simulink model "FOC_sensored"  (R2026a)
settings: Solver=VariableStepAuto  StopTime=3  MaxStep=1e-4  RelTol=1e-4
undefined symbols (not defined in the file): Encoder_resolution, G_filt_back_den_current, G_filt_back_num_current, G_filt_cont_den_current, G_filt_cont_num_current, G_filt_disc_emu_back_den_current, G_filt_disc_emu_back_num_current, G_filt_disc_emu_forw_den_current, G_filt_disc_emu_forw_num_current, G_filt_forw_den_current, G_filt_forw_num_current, In, J, Kr_cont_current, Kr_cont_speed, Kr_direct_back_current, Kr_direct_forw_current, Ld, Lq, Ls, Mn, nn, pp, Psir, T_speed_feedback, Ti_cont_current, Ti_cont_speed, Ti_direct_back_current, Ti_direct_forw_current, Ts_current, Udc
libraries: fl_lib x43, nesl_utility x37, ee_lib x18, eeTransforms x12, slpidlib x5
(part 1 of 2)
settings Model: Creator=LukaPravica  LastModifiedBy=Rio
settings SimscapeCC: ExplicitSolverDiagnosticOptions=none  SimscapeNominalValues="[{\"value\":\"1\",\"unit\":\"A\"},{\"value\":\"1\",\"unit\":\"bar\"},{\"value\":\"1\",\"unit\":\"cm^2\"},{\"value\":\"1\",\"unit\":\"cm^3/s\"},{\"value\":\"1\",\"unit\":\"kJ/kg\"},{\"value\":\"1\",\"unit\":\"kW\"},{\"value\":\"1\",\"unit\":\"l\"},{\"value\":\"1\",\"unit\":\"N\"},{\"value\":\"1\",\"unit\":\"N*m\"},{\"value\":\"1\",\"unit\":\"V\"}]"  SimscapeLogType=none  SimscapeLogDataHistory=5000.0

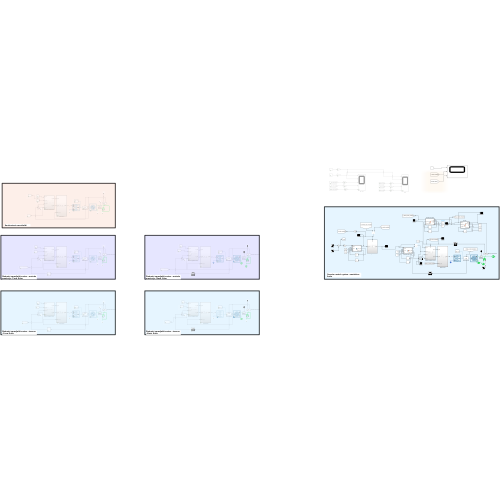
[thumbnail: Simulink's stored preview of the top-level diagram]
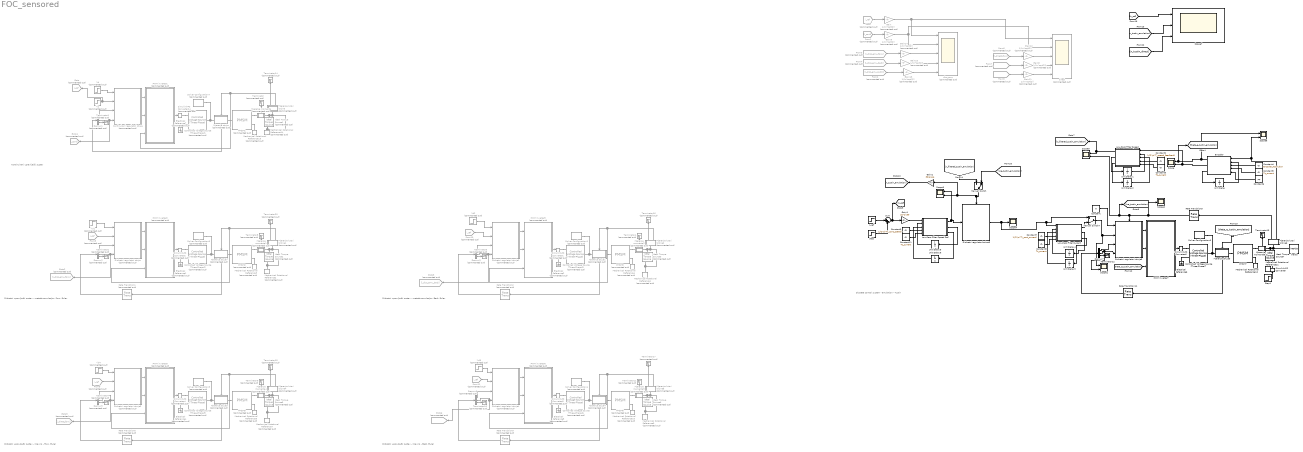
== system FOC_sensored ==
  note: Diskretni upravljački sustav - metoda emulacije - Forw. Euler
  note: Kontinuirani upravljački sustav
  note: Diskretni upravljački sustav - metoda emulacije - Back. Euler
  note: Diskretni upravljački sustav - izravno - Forw. Euler
  note: Diskretni upravljački sustav - izravno - Back. Euler
  note: Discrete control system - emulation - Tustin
  *id{,1..2,4..5} (5 alike) : Step  Commented=on  FinalValue=0  SampleTime=0
  *iq : Step  Commented=on  Time=0.001  FinalValue=In*sqrt(2)  SampleTime=0
  Constant : Constant  Value=0  SampleTime=Ts_current
  Constant{3,5,8,11} (4 alike) : Constant  Value=Ts_current  SampleTime=Ts_current
  Constant2 : Constant  Value=1/(2*pi*T_speed_feedback)  SampleTime=Ts_current
  Constant4 : Constant  Value=Encoder_resolution  SampleTime=Ts_current
  Constant6 : Constant  Value=pp  SampleTime=Ts_current
  Constant7 : Constant  Value=1/(2*pi*Ti_cont_current)  SampleTime=Ts_current
  Constant9 : Constant  Value=1/(2*pi*Ti_cont_speed)  SampleTime=Ts_current
  Controlled Voltage Source (Three-Phase){1..3,5..6} (5 alike) : ee_lib/Sources/Controlled Voltage Source (Three-Phase)  Commented=on  input_option=ee.enum.inputType.instantaneous  FRated=60 Hz
  Controlled Voltage Source (Three-Phase)7 : ee_lib/Sources/Controlled Voltage Source (Three-Phase)  input_option=ee.enum.inputType.instantaneous  FRated=60 Hz
  Demux{1..3,5..6} (5 alike) : Demux  Commented=on  Outputs=3
  Demux7 : Demux  Outputs=3
  Diskretni regulator brzine5 : Subsystem
      settings: PortSchema="{\"entries\":[{\"content\":{\"sides\":[{\"content\":{\"connectorIds\":[\"In1\"]},\"type\":\"ConnectorPlacement.EquallySpacedRectSide\",\"uuid\":\"a9765fbc-5a4d-474e-be8d-5c320c5f07ca\"},{\"content\":{\"connectorIds\":[\"Out1\"],\"side\":\"RIGHT\"},\"type\":\"ConnectorPlacement.EquallySpacedRectSide\",\"uuid\":\"d113e0d0-4772-4877-8676-69342ee8f64f\"},{\"content\":{\"connectorIds\":[\"In2\"],\"side\":\"TOP\"},\"type\":\"ConnectorPlacement.EquallySpacedRectSide\",\"uuid\":\"4ca0dc59-fd41-4846-82a7-6904cf53659d\"}]},\"type\":\"ConnectorPlacement.EquallySpacedConnector\",\"uuid\":\"7fdfac1a-ebdc-43ed-9adb-be729266989d\"}],\"packageUris\":[\"http://schema.mathworks.com/mf0/Connector/R2020b\"],\"version\":\"1.0\"}"
  Diskretni regulatori struje : Subsystem  Commented=on
  Diskretni regulatori struje1 : Subsystem  Commented=on
  Diskretni regulatori struje3 : Subsystem  Commented=on
  Diskretni regulatori struje4 : Subsystem  Commented=on
  Diskretni regulatori struje5 : Subsystem
      settings: PortSchema="{\"entries\":[{\"content\":{\"sides\":[{\"content\":{\"connectorIds\":[\"In1\",\"In2\",\"In3\",\"In4\"]},\"type\":\"ConnectorPlacement.EquallySpacedRectSide\",\"uuid\":\"d3a62493-f7c6-444f-9476-25937989f6ea\"},{\"content\":{\"connectorIds\":[\"Out1\",\"Out2\"],\"side\":\"RIGHT\"},\"type\":\"ConnectorPlacement.EquallySpacedRectSide\",\"uuid\":\"ca5c9823-b9be-4b72-ab87-a2cad855a0f6\"},{\"content\":{\"connectorIds\":[\"In5\"],\"side\":\"TOP\"},\"type\":\"ConnectorPlacement.EquallySpacedRectSide\",\"uuid\":\"496b345e-fed9-4adb-95d9-010d07f11d94\"}]},\"type\":\"ConnectorPlacement.EquallySpacedConnector\",\"uuid\":\"9eb14200-6fae-48ad-9447-ab4bb77ea536\"}],\"packageUris\":[\"http://schema.mathworks.com/mf0/Connector/R2020b\"],\"version\":\"1.0\"}"
  Electrical Reference{1..2,4..5,7} (5 alike) : fl_lib/Electrical/Electrical Elements/Electrical Reference  Commented=on
  Electrical Reference6 : fl_lib/Electrical/Electrical Elements/Electrical Reference
  Encoder : MATLAB Function  TreatAsAtomicUnit=on
  From{,8..11} (5 alike) : From  Commented=on  GotoTag=i_ref  TagVisibility=global
  From1 : From  Commented=on  GotoTag=i_cont
  From2 : From  Commented=on  GotoTag=i_disc_emu_tustin
  From3 : From  Commented=on  GotoTag=i_disc_emu_forw
  From4 : From  Commented=on  GotoTag=i_disc_emu_back
  From5 : From  Commented=on  GotoTag=i_direct_tustin
  From6 : From  Commented=on  GotoTag=i_direct_forw
  From7 : From  Commented=on  GotoTag=i_direct_back
  Gain{,8..14} (8 alike) : Gain  Commented=on  Gain=1/(In*sqrt(2))
  Gain1 : Gain  Gain=pp*pi/30
  Gain2 : Gain  Gain=30/pi/pp
  Goto : Goto  Commented=on  GotoTag=i_ref  TagVisibility=global
  Goto1 : Goto  Commented=on  GotoTag=i_cont
  Goto2 : Goto  Commented=on  GotoTag=i_disc_emu_forw
  Goto3 : Goto  Commented=on  GotoTag=i_disc_emu_back
  Goto5 : Goto  Commented=on  GotoTag=i_direct_forw
  Goto6 : Goto  Commented=on  GotoTag=i_direct_back
  Ideal Torque Source{1..3,5..6} (5 alike) : fl_lib/Mechanical/Mechanical Sources/Ideal Torque Source  Commented=on
  Ideal Torque Source7 : fl_lib/Mechanical/Mechanical Sources/Ideal Torque Source
  Inertia : fl_lib/Mechanical/Rotational Elements/Inertia  inertia=J kg*m^2  num_ports=foundation.enum.numPorts2.one  w_specify=off  w_priority=High  w=0 rad/s  w_nominal_specify=off  w_nominal_value=1  w_nominal_unit=rad/s  t_specify=off  t_priority=None  t=0 N*m  t_nominal_specify=off  t_nominal_value=1  t_nominal_unit=N*m
  Kontinuirani regulatori struje : Subsystem  Commented=on
  Low-Pass Filter Current : MATLAB Function  TreatAsAtomicUnit=on
  Low-Pass Filter Speed : MATLAB Function  TreatAsAtomicUnit=on
  Low-Pass Filter Speed Ref : MATLAB Function  TreatAsAtomicUnit=on
  Manual Switch : ManualSwitch  CurrentSetting=0
  Manual Switch7 : ManualSwitch  CurrentSetting=0
  Mechanical Rotational Reference{1..4,7..10,14..15} (10 alike) : fl_lib/Mechanical/Rotational Elements/Mechanical Rotational Reference  Commented=on
  Mechanical Rotational Reference11 : fl_lib/Mechanical/Rotational Elements/Mechanical Rotational Reference
  Mechanical Rotational Reference12 : fl_lib/Mechanical/Rotational Elements/Mechanical Rotational Reference
  Mjerenje momenta : Subsystem  Commented=on
      settings: PortSchema="{\"entries\":[{\"content\":{\"sides\":[{\"content\":{\"connectorIds\":[\"LConn1\"]},\"type\":\"ConnectorPlacement.EquallySpacedRectSide\",\"uuid\":\"6fa7c16c-6de5-49c8-bc22-739ef8014510\"},{\"content\":{\"connectorIds\":[\"RConn1\"],\"side\":\"RIGHT\"},\"type\":\"ConnectorPlacement.EquallySpacedRectSide\",\"uuid\":\"6cbb3fe1-95dc-4f03-932b-ab8cb637a208\"},{\"content\":{\"connectorIds\":[\"Out1\"],\"side\":\"TOP\"},\"type\":\"ConnectorPlacement.EquallySpacedRectSide\",\"uuid\":\"35a7ae71-901f-47d3-ac0b-d21c2464290d\"}]},\"type\":\"ConnectorPlacement.EquallySpacedConnector\",\"uuid\":\"03aa7740-1fdb-47bb-9a21-844669f6bcda\"}],\"packageUris\":[\"http://schema.mathworks.com/mf0/Connector/R2020b\"],\"version\":\"1.0\"}"
      mask Display: disp('trq')
  Mjerenje momenta1 : Subsystem  Commented=on
      settings: PortSchema="{\"entries\":[{\"content\":{\"sides\":[{\"content\":{\"connectorIds\":[\"LConn1\"]},\"type\":\"ConnectorPlacement.EquallySpacedRectSide\",\"uuid\":\"6fa7c16c-6de5-49c8-bc22-739ef8014510\"},{\"content\":{\"connectorIds\":[\"RConn1\"],\"side\":\"RIGHT\"},\"type\":\"ConnectorPlacement.EquallySpacedRectSide\",\"uuid\":\"6cbb3fe1-95dc-4f03-932b-ab8cb637a208\"},{\"content\":{\"connectorIds\":[\"Out1\"],\"side\":\"TOP\"},\"type\":\"ConnectorPlacement.EquallySpacedRectSide\",\"uuid\":\"35a7ae71-901f-47d3-ac0b-d21c2464290d\"}]},\"type\":\"ConnectorPlacement.EquallySpacedConnector\",\"uuid\":\"03aa7740-1fdb-47bb-9a21-844669f6bcda\"}],\"packageUris\":[\"http://schema.mathworks.com/mf0/Connector/R2020b\"],\"version\":\"1.0\"}"
      mask Display: disp('trq')
  Mjerenje momenta2 : Subsystem  Commented=on
      settings: PortSchema="{\"entries\":[{\"content\":{\"sides\":[{\"content\":{\"connectorIds\":[\"LConn1\"]},\"type\":\"ConnectorPlacement.EquallySpacedRectSide\",\"uuid\":\"6fa7c16c-6de5-49c8-bc22-739ef8014510\"},{\"content\":{\"connectorIds\":[\"RConn1\"],\"side\":\"RIGHT\"},\"type\":\"ConnectorPlacement.EquallySpacedRectSide\",\"uuid\":\"6cbb3fe1-95dc-4f03-932b-ab8cb637a208\"},{\"content\":{\"connectorIds\":[\"Out1\"],\"side\":\"TOP\"},\"type\":\"ConnectorPlacement.EquallySpacedRectSide\",\"uuid\":\"35a7ae71-901f-47d3-ac0b-d21c2464290d\"}]},\"type\":\"ConnectorPlacement.EquallySpacedConnector\",\"uuid\":\"03aa7740-1fdb-47bb-9a21-844669f6bcda\"}],\"packageUris\":[\"http://schema.mathworks.com/mf0/Connector/R2020b\"],\"version\":\"1.0\"}"
      mask Display: disp('trq')
  Mjerenje momenta4 : Subsystem  Commented=on
      settings: PortSchema="{\"entries\":[{\"content\":{\"sides\":[{\"content\":{\"connectorIds\":[\"LConn1\"]},\"type\":\"ConnectorPlacement.EquallySpacedRectSide\",\"uuid\":\"6fa7c16c-6de5-49c8-bc22-739ef8014510\"},{\"content\":{\"connectorIds\":[\"RConn1\"],\"side\":\"RIGHT\"},\"type\":\"ConnectorPlacement.EquallySpacedRectSide\",\"uuid\":\"6cbb3fe1-95dc-4f03-932b-ab8cb637a208\"},{\"content\":{\"connectorIds\":[\"Out1\"],\"side\":\"TOP\"},\"type\":\"ConnectorPlacement.EquallySpacedRectSide\",\"uuid\":\"35a7ae71-901f-47d3-ac0b-d21c2464290d\"}]},\"type\":\"ConnectorPlacement.EquallySpacedConnector\",\"uuid\":\"03aa7740-1fdb-47bb-9a21-844669f6bcda\"}],\"packageUris\":[\"http://schema.mathworks.com/mf0/Connector/R2020b\"],\"version\":\"1.0\"}"
      mask Display: disp('trq')
  Mjerenje momenta5 : Subsystem  Commented=on
      settings: PortSchema="{\"entries\":[{\"content\":{\"sides\":[{\"content\":{\"connectorIds\":[\"LConn1\"]},\"type\":\"ConnectorPlacement.EquallySpacedRectSide\",\"uuid\":\"6fa7c16c-6de5-49c8-bc22-739ef8014510\"},{\"content\":{\"connectorIds\":[\"RConn1\"],\"side\":\"RIGHT\"},\"type\":\"ConnectorPlacement.EquallySpacedRectSide\",\"uuid\":\"6cbb3fe1-95dc-4f03-932b-ab8cb637a208\"},{\"content\":{\"connectorIds\":[\"Out1\"],\"side\":\"TOP\"},\"type\":\"ConnectorPlacement.EquallySpacedRectSide\",\"uuid\":\"35a7ae71-901f-47d3-ac0b-d21c2464290d\"}]},\"type\":\"ConnectorPlacement.EquallySpacedConnector\",\"uuid\":\"03aa7740-1fdb-47bb-9a21-844669f6bcda\"}],\"packageUris\":[\"http://schema.mathworks.com/mf0/Connector/R2020b\"],\"version\":\"1.0\"}"
      mask Display: disp('trq')
  Mjerenje momenta6 : Subsystem
      settings: PortSchema="{\"entries\":[{\"content\":{\"sides\":[{\"content\":{\"connectorIds\":[\"LConn1\"]},\"type\":\"ConnectorPlacement.EquallySpacedRectSide\",\"uuid\":\"6fa7c16c-6de5-49c8-bc22-739ef8014510\"},{\"content\":{\"connectorIds\":[\"RConn1\"],\"side\":\"RIGHT\"},\"type\":\"ConnectorPlacement.EquallySpacedRectSide\",\"uuid\":\"6cbb3fe1-95dc-4f03-932b-ab8cb637a208\"},{\"content\":{\"connectorIds\":[\"Out1\"],\"side\":\"TOP\"},\"type\":\"ConnectorPlacement.EquallySpacedRectSide\",\"uuid\":\"35a7ae71-901f-47d3-ac0b-d21c2464290d\"}]},\"type\":\"ConnectorPlacement.EquallySpacedConnector\",\"uuid\":\"03aa7740-1fdb-47bb-9a21-844669f6bcda\"}],\"packageUris\":[\"http://schema.mathworks.com/mf0/Connector/R2020b\"],\"version\":\"1.0\"}"
      mask Display: disp('trq')
  Mjerenje kuta i brzine : Subsystem  Commented=on
      mask Display: disp('w,a')
  Mjerenje kuta i brzine1 : Subsystem  Commented=on
      mask Display: disp('w,a')
  Mjerenje kuta i brzine2 : Subsystem  Commented=on
      mask Display: disp('w,a')
  Mjerenje kuta i brzine4 : Subsystem  Commented=on
      mask Display: disp('w,a')
  Mjerenje kuta i brzine5 : Subsystem  Commented=on
      mask Display: disp('w,a')
  Mjerenje kuta i brzine6 : Subsystem
      mask Display: disp('w,a')
  Mjerenje struje : Subsystem  Commented=on
      settings: PortSchema="{\"entries\":[{\"content\":{\"sides\":[{\"content\":{\"connectorIds\":[\"LConn1\"]},\"type\":\"ConnectorPlacement.EquallySpacedRectSide\",\"uuid\":\"6fa7c16c-6de5-49c8-bc22-739ef8014510\"},{\"content\":{\"connectorIds\":[\"RConn1\"],\"side\":\"RIGHT\"},\"type\":\"ConnectorPlacement.EquallySpacedRectSide\",\"uuid\":\"6cbb3fe1-95dc-4f03-932b-ab8cb637a208\"},{\"content\":{\"connectorIds\":[\"In1\"],\"side\":\"TOP\"},\"type\":\"ConnectorPlacement.EquallySpacedRectSide\",\"uuid\":\"35a7ae71-901f-47d3-ac0b-d21c2464290d\"},{\"content\":{\"connectorIds\":[\"Out1\"],\"side\":\"BOTTOM\"},\"type\":\"ConnectorPlacement.EquallySpacedRectSide\",\"uuid\":\"976aabfd-697c-47ce-8be7-acff7370fc8c\"}]},\"type\":\"ConnectorPlacement.EquallySpacedConnector\",\"uuid\":\"03aa7740-1fdb-47bb-9a21-844669f6bcda\"}],\"packageUris\":[\"http://schema.mathworks.com/mf0/Connector/R2020b\"],\"version\":\"1.0\"}"
      mask Display: disp('vi abc')
  Mjerenje struje1 : Subsystem  Commented=on
      settings: PortSchema="{\"entries\":[{\"content\":{\"sides\":[{\"content\":{\"connectorIds\":[\"LConn1\"]},\"type\":\"ConnectorPlacement.EquallySpacedRectSide\",\"uuid\":\"6fa7c16c-6de5-49c8-bc22-739ef8014510\"},{\"content\":{\"connectorIds\":[\"RConn1\"],\"side\":\"RIGHT\"},\"type\":\"ConnectorPlacement.EquallySpacedRectSide\",\"uuid\":\"6cbb3fe1-95dc-4f03-932b-ab8cb637a208\"},{\"content\":{\"connectorIds\":[\"In1\"],\"side\":\"TOP\"},\"type\":\"ConnectorPlacement.EquallySpacedRectSide\",\"uuid\":\"35a7ae71-901f-47d3-ac0b-d21c2464290d\"},{\"content\":{\"connectorIds\":[\"Out1\"],\"side\":\"BOTTOM\"},\"type\":\"ConnectorPlacement.EquallySpacedRectSide\",\"uuid\":\"976aabfd-697c-47ce-8be7-acff7370fc8c\"}]},\"type\":\"ConnectorPlacement.EquallySpacedConnector\",\"uuid\":\"03aa7740-1fdb-47bb-9a21-844669f6bcda\"}],\"packageUris\":[\"http://schema.mathworks.com/mf0/Connector/R2020b\"],\"version\":\"1.0\"}"
      mask Display: disp('vi abc')
  Mjerenje struje3 : Subsystem  Commented=on
      settings: PortSchema="{\"entries\":[{\"content\":{\"sides\":[{\"content\":{\"connectorIds\":[\"LConn1\"]},\"type\":\"ConnectorPlacement.EquallySpacedRectSide\",\"uuid\":\"6fa7c16c-6de5-49c8-bc22-739ef8014510\"},{\"content\":{\"connectorIds\":[\"RConn1\"],\"side\":\"RIGHT\"},\"type\":\"ConnectorPlacement.EquallySpacedRectSide\",\"uuid\":\"6cbb3fe1-95dc-4f03-932b-ab8cb637a208\"},{\"content\":{\"connectorIds\":[\"In1\"],\"side\":\"TOP\"},\"type\":\"ConnectorPlacement.EquallySpacedRectSide\",\"uuid\":\"35a7ae71-901f-47d3-ac0b-d21c2464290d\"},{\"content\":{\"connectorIds\":[\"Out1\"],\"side\":\"BOTTOM\"},\"type\":\"ConnectorPlacement.EquallySpacedRectSide\",\"uuid\":\"976aabfd-697c-47ce-8be7-acff7370fc8c\"}]},\"type\":\"ConnectorPlacement.EquallySpacedConnector\",\"uuid\":\"03aa7740-1fdb-47bb-9a21-844669f6bcda\"}],\"packageUris\":[\"http://schema.mathworks.com/mf0/Connector/R2020b\"],\"version\":\"1.0\"}"
      mask Display: disp('vi abc')
  Mjerenje struje4 : Subsystem  Commented=on
      settings: PortSchema="{\"entries\":[{\"content\":{\"sides\":[{\"content\":{\"connectorIds\":[\"LConn1\"]},\"type\":\"ConnectorPlacement.EquallySpacedRectSide\",\"uuid\":\"6fa7c16c-6de5-49c8-bc22-739ef8014510\"},{\"content\":{\"connectorIds\":[\"RConn1\"],\"side\":\"RIGHT\"},\"type\":\"ConnectorPlacement.EquallySpacedRectSide\",\"uuid\":\"6cbb3fe1-95dc-4f03-932b-ab8cb637a208\"},{\"content\":{\"connectorIds\":[\"In1\"],\"side\":\"TOP\"},\"type\":\"ConnectorPlacement.EquallySpacedRectSide\",\"uuid\":\"35a7ae71-901f-47d3-ac0b-d21c2464290d\"},{\"content\":{\"connectorIds\":[\"Out1\"],\"side\":\"BOTTOM\"},\"type\":\"ConnectorPlacement.EquallySpacedRectSide\",\"uuid\":\"976aabfd-697c-47ce-8be7-acff7370fc8c\"}]},\"type\":\"ConnectorPlacement.EquallySpacedConnector\",\"uuid\":\"03aa7740-1fdb-47bb-9a21-844669f6bcda\"}],\"packageUris\":[\"http://schema.mathworks.com/mf0/Connector/R2020b\"],\"version\":\"1.0\"}"
      mask Display: disp('vi abc')
  Mjerenje struje5 : Subsystem
      settings: PortSchema="{\"entries\":[{\"content\":{\"sides\":[{\"content\":{\"connectorIds\":[\"LConn1\"]},\"type\":\"ConnectorPlacement.EquallySpacedRectSide\",\"uuid\":\"6fa7c16c-6de5-49c8-bc22-739ef8014510\"},{\"content\":{\"connectorIds\":[\"RConn1\"],\"side\":\"RIGHT\"},\"type\":\"ConnectorPlacement.EquallySpacedRectSide\",\"uuid\":\"6cbb3fe1-95dc-4f03-932b-ab8cb637a208\"},{\"content\":{\"connectorIds\":[\"In1\"],\"side\":\"TOP\"},\"type\":\"ConnectorPlacement.EquallySpacedRectSide\",\"uuid\":\"35a7ae71-901f-47d3-ac0b-d21c2464290d\"},{\"content\":{\"connectorIds\":[\"Out1\"],\"side\":\"BOTTOM\"},\"type\":\"ConnectorPlacement.EquallySpacedRectSide\",\"uuid\":\"976aabfd-697c-47ce-8be7-acff7370fc8c\"}]},\"type\":\"ConnectorPlacement.EquallySpacedConnector\",\"uuid\":\"03aa7740-1fdb-47bb-9a21-844669f6bcda\"}],\"packageUris\":[\"http://schema.mathworks.com/mf0/Connector/R2020b\"],\"version\":\"1.0\"}"
      mask Display: disp('vi abc')
  Mjerenje struje7 : Subsystem  Commented=on
      settings: PortSchema="{\"entries\":[{\"content\":{\"sides\":[{\"content\":{\"connectorIds\":[\"LConn1\"]},\"type\":\"ConnectorPlacement.EquallySpacedRectSide\",\"uuid\":\"6fa7c16c-6de5-49c8-bc22-739ef8014510\"},{\"content\":{\"connectorIds\":[\"RConn1\"],\"side\":\"RIGHT\"},\"type\":\"ConnectorPlacement.EquallySpacedRectSide\",\"uuid\":\"6cbb3fe1-95dc-4f03-932b-ab8cb637a208\"},{\"content\":{\"connectorIds\":[\"In1\"],\"side\":\"TOP\"},\"type\":\"ConnectorPlacement.EquallySpacedRectSide\",\"uuid\":\"35a7ae71-901f-47d3-ac0b-d21c2464290d\"},{\"content\":{\"connectorIds\":[\"Out1\"],\"side\":\"BOTTOM\"},\"type\":\"ConnectorPlacement.EquallySpacedRectSide\",\"uuid\":\"976aabfd-697c-47ce-8be7-acff7370fc8c\"}]},\"type\":\"ConnectorPlacement.EquallySpacedConnector\",\"uuid\":\"03aa7740-1fdb-47bb-9a21-844669f6bcda\"}],\"packageUris\":[\"http://schema.mathworks.com/mf0/Connector/R2020b\"],\"version\":\"1.0\"}"
      mask Display: disp('vi abc')
  PMSM1 : ee_lib/Electromechanical/Permanent Magnet/PMSM  Commented=on  port_option=ee.enum.threePhasePort.composite  winding_type=ee.enum.statorconnection.wye  machine_param=ee.enum.pmsm.parameterization.constant  nPolePairs=pp  pmflux_param=ee.enum.pmflux.fluxlinkage  pm_flux_linkage=Psir Wb  torque_constant=0.18 N*m/A  back_emf_constant=0.18 V/rpm  stator_param=ee.enum.statorparam.LdLqL0  Ld=Ls H  Lq=Ls H  idVec=[-200, 0, 200] A  iqVec=[-200, 0, 200] A  LdMatrix=0.0002 * ones(3, 3) H  LqMatrix=0.0002 * ones(3, 3) H  PmMatrix=0.1 * ones(3, 3) Wb  ktMatrix=0.18 * ones(3, 3) N*m/A  keMatrix=0.18 * ones(3, 3) V*s/rad  L0=(Ld+Lq)/2 H  Ls=0.0002 H  Lm=-0.00002 H  Ms=0.00002 H  Rs=Rs Ohm  zero_sequence=ee.enum.park.zerosequence.exclude  axes_param=ee.enum.rotorangle.daxis  loss_param=ee.enum.ironloss.none  losses_oc=[0, 0, 0] W  losses_sc=[0, 0, 0] W  f_losses=60 Hz  Isc_losses=95 A  J=J kg*m^2  lam=D N*m*s/rad  i_d_specify=off  i_d_priority=None  i_d=0 A  i_d_nominal_specify=off  i_d_nominal_value=1  i_d_nominal_unit=A  i_q_specify=off  i_q_priority=None  i_q=0 A  i_q_nominal_specify=off  i_q_nominal_value=1  i_q_nominal_unit=A  torque_specify=off  torque_priority=None  torque=0 N*m  torque_nominal_specify=off  torque_nominal_value=1  torque_nominal_unit=N*m  angular_velocity_specify=off  angular_velocity_priority=High  angular_velocity=0 rpm  angular_velocity_nominal_specify=off  angular_velocity_nominal_value=1  angular_velocity_nominal_unit=rpm  angular_position_specify=off  angular_position_priority=High  angular_position=0 deg  angular_position_nominal_specify=off  angular_position_nominal_value=1  angular_position_nominal_unit=deg  alpha=3.93e-3 1/K  alpha_flux=-0.001 1/K  Tmeas=298.15 K  stator_thermal_mass=100 J/K  rotor_thermal_mass=200 J/K  Rm_percent_rotor=90  Rd_percent_rotor=30  temperatureA_specify=off  temperatureA_priority=High  temperatureA=25 degC  temperatureA_nominal_specify=off  temperatureA_nominal_value=1  temperatureA_nominal_unit=degC  temperatureB_specify=off  temperatureB_priority=High  temperatureB=25 degC  temperatureB_nominal_specify=off  temperatureB_nominal_value=1  temperatureB_nominal_unit=degC  temperatureC_specify=off  temperatureC_priority=High  temperatureC=25 degC  temperatureC_nominal_specify=off  temperatureC_nominal_value=1  temperatureC_nominal_unit=degC  temperatureR_specify=off  temperatureR_priority=High  temperatureR=25 degC  temperatureR_nominal_specify=off  temperatureR_nominal_value=1  temperatureR_nominal_unit=degC
  PMSM{2..3,5..6} (4 alike) : ee_lib/Electromechanical/Permanent Magnet/PMSM  Commented=on  port_option=ee.enum.threePhasePort.composite  winding_type=ee.enum.statorconnection.wye  machine_param=ee.enum.pmsm.parameterization.constant  nPolePairs=pp  pmflux_param=ee.enum.pmflux.fluxlinkage  pm_flux_linkage=Psir Wb  torque_constant=0.18 N*m/A  back_emf_constant=0.18 V*s/rad  stator_param=ee.enum.statorparam.LdLqL0  Ld=Ls H  Lq=Ls H  idVec=[-200, 0, 200] A  iqVec=[-200, 0, 200] A  LdMatrix=0.0002 * ones(3, 3) H  LqMatrix=0.0002 * ones(3, 3) H  PmMatrix=0.1 * ones(3, 3) Wb  ktMatrix=0.18 * ones(3, 3) N*m/A  keMatrix=0.18 * ones(3, 3) V*s/rad  L0=(Ld+Lq)/2 H  Ls=0.0002 H  Lm=-0.00002 H  Ms=0.00002 H  Rs=Rs Ohm  zero_sequence=ee.enum.park.zerosequence.exclude  axes_param=ee.enum.rotorangle.daxis  loss_param=ee.enum.ironloss.none  losses_oc=[0, 0, 0] W  losses_sc=[0, 0, 0] W  f_losses=60 Hz  Isc_losses=95 A  J=J kg*m^2  lam=D N*m*s/rad  i_d_specify=off  i_d_priority=None  i_d=0 A  i_d_nominal_specify=off  i_d_nominal_value=1  i_d_nominal_unit=A  i_q_specify=off  i_q_priority=None  i_q=0 A  i_q_nominal_specify=off  i_q_nominal_value=1  i_q_nominal_unit=A  torque_specify=off  torque_priority=None  torque=0 N*m  torque_nominal_specify=off  torque_nominal_value=1  torque_nominal_unit=N*m  angular_velocity_specify=off  angular_velocity_priority=High  angular_velocity=0 rpm  angular_velocity_nominal_specify=off  angular_velocity_nominal_value=1  angular_velocity_nominal_unit=rpm  angular_position_specify=off  angular_position_priority=High  angular_position=0 deg  angular_position_nominal_specify=off  angular_position_nominal_value=1  angular_position_nominal_unit=deg  alpha=3.93e-3 1/K  alpha_flux=-0.001 1/K  Tmeas=298.15 K  stator_thermal_mass=100 J/K  rotor_thermal_mass=200 J/K  Rm_percent_rotor=90  Rd_percent_rotor=30  temperatureA_specify=off  temperatureA_priority=High  temperatureA=25 degC  temperatureA_nominal_specify=off  temperatureA_nominal_value=1  temperatureA_nominal_unit=degC  temperatureB_specify=off  temperatureB_priority=High  temperatureB=25 degC  temperatureB_nominal_specify=off  temperatureB_nominal_value=1  temperatureB_nominal_unit=degC  temperatureC_specify=off  temperatureC_priority=High  temperatureC=25 degC  temperatureC_nominal_specify=off  temperatureC_nominal_value=1  temperatureC_nominal_unit=degC  temperatureR_specify=off  temperatureR_priority=High  temperatureR=25 degC  temperatureR_nominal_specify=off  temperatureR_nominal_value=1  temperatureR_nominal_unit=degC
  PMSM7 : ee_lib/Electromechanical/Permanent Magnet/PMSM  port_option=ee.enum.threePhasePort.composite  winding_type=ee.enum.statorconnection.wye  machine_param=ee.enum.pmsm.parameterization.constant  nPolePairs=pp  pmflux_param=ee.enum.pmflux.fluxlinkage  pm_flux_linkage=Psir Wb  torque_constant=0.18 N*m/A  back_emf_constant=0.18 V*s/rad  stator_param=ee.enum.statorparam.LdLqL0  Ld=Ls H  Lq=Ls H  idVec=[-200, 0, 200] A  iqVec=[-200, 0, 200] A  LdMatrix=0.0002 * ones(3, 3) H  LqMatrix=0.0002 * ones(3, 3) H  PmMatrix=0.1 * ones(3, 3) Wb  ktMatrix=0.18 * ones(3, 3) N*m/A  keMatrix=0.18 * ones(3, 3) V*s/rad  L0=(Ld+Lq)/2 H  Ls=0.0002 H  Lm=-0.00002 H  Ms=0.00002 H  Rs=Rs Ohm  zero_sequence=ee.enum.park.zerosequence.exclude  axes_param=ee.enum.rotorangle.daxis  loss_param=ee.enum.ironloss.none  losses_oc=[0, 0, 0] W  losses_sc=[0, 0, 0] W  f_losses=60 Hz  Isc_losses=95 A  J=J kg*m^2  lam=D N*m*s/rad  i_d_specify=off  i_d_priority=None  i_d=0 A  i_d_nominal_specify=off  i_d_nominal_value=1  i_d_nominal_unit=A  i_q_specify=off  i_q_priority=High  i_q=7.1 A  i_q_nominal_specify=on  i_q_nominal_value=7.1  i_q_nominal_unit=A  torque_specify=off  torque_priority=None  torque=0 N*m  torque_nominal_specify=on  torque_nominal_value=Mn  torque_nominal_unit=N*m  angular_velocity_specify=off  angular_velocity_priority=High  angular_velocity=0 rpm  angular_velocity_nominal_specify=on  angular_velocity_nominal_value=6000  angular_velocity_nominal_unit=rpm  angular_position_specify=off  angular_position_priority=High  angular_position=0 deg  angular_position_nominal_specify=off  angular_position_nominal_value=1  angular_position_nominal_unit=deg  alpha=3.93e-3 1/K  alpha_flux=-0.001 1/K  Tmeas=298.15 K  stator_thermal_mass=100 J/K  rotor_thermal_mass=200 J/K  Rm_percent_rotor=90  Rd_percent_rotor=30  temperatureA_specify=off  temperatureA_priority=High  temperatureA=25 degC  temperatureA_nominal_specify=off  temperatureA_nominal_value=1  temperatureA_nominal_unit=degC  temperatureB_specify=off  temperatureB_priority=High  temperatureB=25 degC  temperatureB_nominal_specify=off  temperatureB_nominal_value=1  temperatureB_nominal_unit=degC  temperatureC_specify=off  temperatureC_priority=High  temperatureC=25 degC  temperatureC_nominal_specify=off  temperatureC_nominal_value=1  temperatureC_nominal_unit=degC  temperatureR_specify=off  temperatureR_priority=High  temperatureR=25 degC  temperatureR_nominal_specify=off  temperatureR_nominal_value=1  temperatureR_nominal_unit=degC
  PWM inverter1 : Subsystem  Commented=on
  PWM inverter2 : Subsystem  Commented=on
  PWM inverter3 : Subsystem  Commented=on
  PWM inverter5 : Subsystem  Commented=on
  PWM inverter6 : Subsystem  Commented=on
  PWM inverter7 : Subsystem
  Rate Transition{1..2,6,9} (4 alike) : RateTransition  Commented=on  OutPortSampleTime=Ts_current
  Rate Transition11 : RateTransition  OutPortSampleTime=Ts_current
  Rate Transition5 : RateTransition  OutPortSampleTime=Ts_current
  Scope{,1,3,5..6} (5 alike) : Scope  NumInputPorts=2
      Scope settings: ActiveDisplayYMinimum=-375.02762302228257  ActiveDisplayYMaximum=3375.2486072005436
      Scope1 settings: ActiveDisplayYMinimum=-1.2628287030818877  ActiveDisplayYMaximum=12.893717206376554  DataLoggingVariableName=ScopeData6
      Scope3 settings: ActiveDisplayYMinimum=-104.71974768783154  ActiveDisplayYMaximum=942.47772919048418  DataLoggingVariableName=ScopeData8
      Scope5 settings: ActiveDisplayYMinimum=-274.10667777849955  ActiveDisplayYMaximum=2466.9601000064963  DataLoggingVariableName=ScopeData11
      Scope6 settings: ActiveDisplayYMinimum=-0.51413414630907539  ActiveDisplayYMaximum=7.2788214815531873  DataLoggingVariableName=ScopeData12
  Scope2 : Scope
      settings: ActiveDisplayYMinimum=-5281.0613442070317  ActiveDisplayYMaximum=3730.2587788855749  DataLoggingVariableName=ScopeData7
  Scope4 : Scope
      settings: ActiveDisplayYMinimum=-66.335912940720434  ActiveDisplayYMaximum=63.17125095285094  DataLoggingVariableName=ScopeData9
  Scope7 : Scope  NumInputPorts=3
      settings: ActiveDisplayYMinimum=-976.46653495125247  ActiveDisplayYMaximum=2709.4621367034024  DataLoggingVariableName=ScopeData13
  Simulink-PS Converter : nesl_utility/Simulink-PS Converter  PhysicalDomain=network_engine_domain  SubClassName=ps_input  LeftPortType=input  RightPortType=output  PseudoPeriodic=off  Frequencies=[]  NoiseDistribution=none  NoiseParameters=[]  Unit=1  AffineConversion=off  FilteringAndDerivatives=provide  SimscapeFilterOrder=1  InputFilterTimeConstant=0.001  UdotUserProvided=0
  Simulink-PS Converter{1..2,4..5,14} (5 alike) : nesl_utility/Simulink-PS Converter  Commented=on  PhysicalDomain=network_engine_domain  SubClassName=ps_input  LeftPortType=input  RightPortType=output  PseudoPeriodic=off  Frequencies=[]  NoiseDistribution=none  NoiseParameters=[]  Unit=1  AffineConversion=off  FilteringAndDerivatives=provide  SimscapeFilterOrder=1  InputFilterTimeConstant=0.001  UdotUserProvided=0
  Simulink-PS Converter6 : nesl_utility/Simulink-PS Converter  PhysicalDomain=network_engine_domain  SubClassName=ps_input  LeftPortType=input  RightPortType=output  PseudoPeriodic=off  Frequencies=[]  NoiseDistribution=none  NoiseParameters=[]  Unit=1  AffineConversion=off  FilteringAndDerivatives=provide  SimscapeFilterOrder=1  InputFilterTimeConstant=0.001  UdotUserProvided=0
  Solver Configuration{1,3..5,7} (5 alike) : nesl_utility/Solver Configuration  Commented=on  PhysicalDomain=network_engine_domain  SubClassName=solver  LeftPortType=input  RightPortType=generic  Tones=[]  Harmonics=[]  SimulateNoise=off  Profile=off  UseLocalSampling=off  EnableSwitchedLinearOptims=on  FrequencyDomain=off  UseCCode=off  RelTol=0.001  AbsTol=0.001  MinStep=1e-09  ToWorkspace=off  RevertToSquareIcSolve=off  NumHomotopyIterations=100  PhasorMode=off  PhasorModeNumHarmonics=1  ConsistencySolver=NEWTON_XTOL_AFTER_FTOL  CanonicalOrdering=UNORDERED  OptimizeIntermediates=UNOPTIMIZED  IndexReductionMethod=DerivativeReplacement  DoDC=off  ResidualTolerance=1e-09  ConsistencyTolSource=GLOBAL  ConsistencyAbsTol=0.001  ConsistencyRelTol=0.001  ConsistencyTolFactor=0.001  UseLocalSolver=off  LocalSolverChoice=NE_BACKWARD_EULER_ADVANCER  ResolveIndetEquations=on  FunctionEvalNumThread=1  LocalSolverSampleTime=0.001  DoFixedCost=off  MaxNonlinIter=3  MaxModeIter=2  ComputeImpulses=off  ImpulseIterations=2  LinearAlgebra=auto  LinearAlgebraNumThread=0  EquationFormulation=NE_TIME_EF  DelaysMemoryBudget=1024  AutomaticFiltering=on  FilteringTimeConstant=0.001  PartitionStorageMethod=AS_NEEDED  PartitionMemoryBudget=1024  PartitionMethod=ROBUST  MultibodyUseLocalSolver=off  MultibodyLocalSolverChoice=ODE1  MultibodyLocalSolverSampleTime=0.001
  Solver Configuration6 : nesl_utility/Solver Configuration  PhysicalDomain=network_engine_domain  SubClassName=solver  LeftPortType=input  RightPortType=generic  Tones=[]  Harmonics=[]  SimulateNoise=off  Profile=off  UseLocalSampling=off  EnableSwitchedLinearOptims=on  FrequencyDomain=off  UseCCode=off  RelTol=0.001  AbsTol=0.001  MinStep=1e-09  ToWorkspace=off  RevertToSquareIcSolve=off  NumHomotopyIterations=100  PhasorMode=off  PhasorModeNumHarmonics=1  ConsistencySolver=NEWTON_XTOL_AFTER_FTOL  CanonicalOrdering=UNORDERED  OptimizeIntermediates=UNOPTIMIZED  IndexReductionMethod=DerivativeReplacement  DoDC=off  ResidualTolerance=1e-09  ConsistencyTolSource=GLOBAL  ConsistencyAbsTol=0.001  ConsistencyRelTol=0.001  ConsistencyTolFactor=0.001  UseLocalSolver=off  LocalSolverChoice=NE_BACKWARD_EULER_ADVANCER  ResolveIndetEquations=on  FunctionEvalNumThread=1  LocalSolverSampleTime=0.001  DoFixedCost=off  MaxNonlinIter=3  MaxModeIter=2  ComputeImpulses=off  ImpulseIterations=2  LinearAlgebra=auto  LinearAlgebraNumThread=0  EquationFormulation=NE_TIME_EF  DelaysMemoryBudget=1024  AutomaticFiltering=on  FilteringTimeConstant=0.001  PartitionStorageMethod=AS_NEEDED  PartitionMemoryBudget=1024  PartitionMethod=ROBUST  MultibodyUseLocalSolver=off  MultibodyLocalSolverChoice=ODE1  MultibodyLocalSolverSampleTime=0.001
  Step : Step  Time=0.5  FinalValue=-1200  SampleTime=0
  Step1 : Step  Time=1.5  FinalValue=-Mn/2  SampleTime=0
  Sum : Sum  Inputs=|++
  Terminator{,1..4,7..11,14..17,20} (15 alike) : Terminator  Commented=on
  Terminator12 : Terminator
  Terminator13 : Terminator
  Unit Delay{,1..6} (7 alike) : UnitDelay  SampleTime=Ts_current
  direct : Scope  Commented=on  NumInputPorts=5
      settings: ActiveDisplayYMinimum=-0.16896  ActiveDisplayYMaximum=1.52065  DataLoggingVariableName=ScopeData2
  disc_emu : Scope  Commented=on  NumInputPorts=5
      settings: ActiveDisplayYMinimum=0.8587  ActiveDisplayYMaximum=1.49811  DataLoggingVariableName=ScopeData3
  n_ref : Step  Time=0.1  FinalValue=2000  SampleTime=0
  wires:
  Demux1/3 -> Terminator1/1
  Demux1/1 -> Kontinuirani regulatori struje/3(id_mj)
  Kontinuirani regulatori struje/1(ud_ref) -> PWM inverter1/1(ud_ref)
  Demux1/2 -> Goto1/1, Kontinuirani regulatori struje/4(iq_mj)
  PWM inverter1/1(u_abc*) -> Simulink-PS Converter14/1
  Mjerenje kuta i brzine/2(Output1) -> PWM inverter1/3(theta_e_mj), Mjerenje struje/1(Input)
  Kontinuirani regulatori struje/2(uq_ref) -> PWM inverter1/2(uq_ref)
  PWM inverter2/1(u_abc*) -> Simulink-PS Converter2/1
  Demux2/3 -> Terminator2/1
  Demux2/1 -> Diskretni regulatori struje/3(id_mj)
  Demux2/2 -> Goto2/1, Diskretni regulatori struje/4(iq_mj)
  Diskretni regulatori struje/1(ud_ref) -> PWM inverter2/1(ud_ref)
  Diskretni regulatori struje/2(uq_ref) -> PWM inverter2/2(uq_ref)
  Rate Transition1/1 -> Demux2/1
  Mjerenje struje7/1(Output) -> Rate Transition1/1
  Mjerenje struje/1(Output) -> Demux1/1
  Mjerenje momenta/1(Output) -> Terminator/1
  Mjerenje momenta1/1(Output) -> Terminator8/1
  Mjerenje kuta i brzine1/2(Output1) -> Mjerenje struje7/1(Input), PWM inverter2/3(theta_e_mj)
  *iq/1 -> Kontinuirani regulatori struje/2(iq_ref), Goto/1
  *id/1 -> Kontinuirani regulatori struje/1(id_ref)
  Diskretni regulatori struje1/2(uq_ref) -> PWM inverter3/2(uq_ref)
  Demux3/2 -> Goto3/1, Diskretni regulatori struje1/4(iq_mj)
  Rate Transition2/1 -> Demux3/1
  PWM inverter3/1(u_abc*) -> Simulink-PS Converter1/1
  Demux3/1 -> Diskretni regulatori struje1/3(id_mj)
  Mjerenje kuta i brzine2/2(Output1) -> Mjerenje struje1/1(Input), PWM inverter3/3(theta_e_mj)
  Demux3/3 -> Terminator3/1
  Mjerenje momenta2/1(Output) -> Terminator4/1
  Mjerenje struje1/1(Output) -> Rate Transition2/1
  Diskretni regulatori struje3/2(uq_ref) -> PWM inverter5/2(uq_ref)
  Demux5/2 -> Diskretni regulatori struje3/4(iq_mj), Goto5/1
  Rate Transition6/1 -> Demux5/1
  PWM inverter5/1(u_abc*) -> Simulink-PS Converter4/1
  Demux5/1 -> Diskretni regulatori struje3/3(id_mj)
  Mjerenje kuta i brzine4/2(Output1) -> Mjerenje struje3/1(Input), PWM inverter5/3(theta_e_mj)
  Diskretni regulatori struje3/1(ud_ref) -> PWM inverter5/1(ud_ref)
  Demux5/3 -> Terminator7/1
  Mjerenje momenta4/1(Output) -> Terminator9/1
  Mjerenje struje3/1(Output) -> Rate Transition6/1
  Diskretni regulatori struje4/2(uq_ref) -> PWM inverter6/2(uq_ref)
  Demux6/2 -> Goto6/1, Diskretni regulatori struje4/4(iq_mj)
  Rate Transition9/1 -> Demux6/1
  PWM inverter6/1(u_abc*) -> Simulink-PS Converter5/1
  Demux6/1 -> Diskretni regulatori struje4/3(id_mj)
  Mjerenje kuta i brzine5/2(Output1) -> Mjerenje struje4/1(Input), PWM inverter6/3(theta_e_mj)
  Diskretni regulatori struje4/1(ud_ref) -> PWM inverter6/1(ud_ref)
  Demux6/3 -> Terminator10/1
  Mjerenje momenta5/1(Output) -> Terminator11/1
  Mjerenje struje4/1(Output) -> Rate Transition9/1
  Diskretni regulatori struje5/2(uq_ref) -> PWM inverter7/2(uq_ref)
  Demux7/2 -> Scope1/2, Diskretni regulatori struje5/4(iq_mj)
  Rate Transition11/1 -> Demux7/1
  PWM inverter7/1(u_abc*) -> Simulink-PS Converter6/1
  Demux7/1 -> Diskretni regulatori struje5/3(id_mj)
  Mjerenje kuta i brzine6/2(theta_e) -> Scope6/2, Encoder/1(angle)
  Diskretni regulatori struje5/1(ud_ref) -> PWM inverter7/1(ud_ref)
  Demux7/3 -> Terminator12/1
  Mjerenje momenta6/1(Output) -> Terminator13/1
  Mjerenje struje5/1(Output) -> Rate Transition11/1
  *id1/1 -> Diskretni regulatori struje/1(id_ref)
  Diskretni regulatori struje1/1(ud_ref) -> PWM inverter3/1(ud_ref)
  *id2/1 -> Diskretni regulatori struje1/1(id_ref)
  From10/1 -> Diskretni regulatori struje1/2(iq_ref)
  *id4/1 -> Diskretni regulatori struje3/1(id_ref)
  From9/1 -> Diskretni regulatori struje3/2(iq_ref)
  *id5/1 -> Diskretni regulatori struje4/1(id_ref)
  From11/1 -> Diskretni regulatori struje4/2(iq_ref)
  Mjerenje kuta i brzine/1(Output) -> Terminator14/1
  Mjerenje kuta i brzine4/1(Output) -> Terminator15/1
  Mjerenje kuta i brzine2/1(Output) -> Terminator16/1
  Mjerenje kuta i brzine5/1(Output) -> Terminator17/1
  Mjerenje kuta i brzine6/1(we) -> Rate Transition5/1
  Mjerenje kuta i brzine1/1(Output) -> Terminator20/1
  Gain9/1 -> disc_emu/2, direct/2
  From7/1 -> Gain8/1
  From1/1 -> Gain9/1
  From2/1 -> Gain13/1
  Gain14/1 -> disc_emu/3
  From4/1 -> Gain10/1
  Gain11/1 -> direct/5
  From3/1 -> Gain14/1
  Gain13/1 -> disc_emu/5
  Gain8/1 -> direct/4
  From/1 -> Gain/1
  From6/1 -> Gain12/1
  Gain12/1 -> direct/3
  Gain/1 -> direct/1, disc_emu/1
  From5/1 -> Gain11/1
  Gain10/1 -> disc_emu/4
  From8/1 -> Diskretni regulatori struje/2(iq_ref)
  Rate Transition5/1 -> Scope2/1, [we_tustin_emulation], Scope5/2, Diskretni regulatori struje5/5(we)
  Unit Delay/1 -> Encoder/2(angle_prev)
  Encoder/3(q_angle) -> Unit Delay/1
  Constant/1 -> Diskretni regulatori struje5/1(id_ref)
  Encoder/1(theta_e) -> Scope6/1, [theta_e_tustin_emulation], Scope/1
  Encoder/2(omega_e) -> Low-Pass Filter Speed/1(x), Scope/2
  Low-Pass Filter Speed/2(y_prev_out) -> Unit Delay1/1
  Unit Delay1/1 -> Low-Pass Filter Speed/2(y_prev)
  Low-Pass Filter Speed/1(y) -> [w_filtered_tustin_emulation], Scope5/1
  Low-Pass Filter Speed/3(x_prev_out) -> Unit Delay2/1
  Unit Delay2/1 -> Low-Pass Filter Speed/3(x_prev)
  Step/1 -> Sum/2
  Diskretni regulator brzine5/1(iq_ref) -> Low-Pass Filter Current/1(x), Manual Switch7/1, Scope4/1
  Manual Switch7/1 -> Scope1/1, Diskretni regulatori struje5/2(iq_ref)
  Low-Pass Filter Current/1(y) -> Manual Switch7/2
  Low-Pass Filter Current/2(y_prev_out) -> Unit Delay4/1
  Unit Delay4/1 -> Low-Pass Filter Current/2(y_prev)
  Low-Pass Filter Current/3(x_prev_out) -> Unit Delay3/1
  Unit Delay3/1 -> Low-Pass Filter Current/3(x_prev)
  Sum/1 -> [n_ref], Gain1/1
  n_ref/1 -> Sum/1
  Gain1/1 -> Low-Pass Filter Speed Ref/1(x)
  Low-Pass Filter Speed Ref/1(y) -> Scope3/1, Diskretni regulator brzine5/1(w_ref)
  Low-Pass Filter Speed Ref/2(y_prev_out) -> Unit Delay5/1
  Unit Delay5/1 -> Low-Pass Filter Speed Ref/2(y_prev)
  Low-Pass Filter Speed Ref/3(x_prev_out) -> Unit Delay6/1
  Unit Delay6/1 -> Low-Pass Filter Speed Ref/3(x_prev)
  Step1/1 -> Simulink-PS Converter/1
  Manual Switch/1 -> Diskretni regulator brzine5/2(w_mj), Gain2/1, Scope3/2
  [w_filtered_tustin_emulation] -> Manual Switch/1
  [we_tustin_emulation] -> Manual Switch/2
  [theta_e_tustin_emulation] -> Mjerenje struje5/1(Input)
  [theta_e_tustin_emulation] -> PWM inverter7/3(theta_e_mj)
  Constant2/1 -> Low-Pass Filter Speed/4(fc)
  Constant3/1 -> Low-Pass Filter Speed/5(TS)
  Constant4/1 -> Encoder/3(N)
  Constant5/1 -> Encoder/4(dt)
  Constant6/1 -> Encoder/5(pole_pairs)
  Constant7/1 -> Low-Pass Filter Current/4(fc)
  Constant8/1 -> Low-Pass Filter Current/5(TS)
  Constant9/1 -> Low-Pass Filter Speed Ref/4(fc)
  Constant11/1 -> Low-Pass Filter Speed Ref/5(TS)
  Gain2/1 -> [n_tustin_emulation]
  [n_ref] -> Scope7/1
  [n_tustin_emulation] -> Scope7/2
  [n_tustin_direct] -> Scope7/3
  connections:
  Controlled Voltage Source (Three-Phase)1/RConn1 -- Solver Configuration7/RConn1 -- Mjerenje struje/LConn1
  PMSM1/RConn1 -- Mjerenje momenta/LConn1
  Mjerenje momenta/RConn1 -- Ideal Torque Source1/RConn2 -- Mechanical Rotational Reference14/LConn1 -- Mjerenje kuta i brzine/LConn1 -- Ideal Torque Source1/LConn1
  Electrical Reference7/LConn1 -- Controlled Voltage Source (Three-Phase)1/LConn2
  PMSM1/LConn1 -- Mjerenje struje/RConn1
  Simulink-PS Converter14/RConn1 -- Controlled Voltage Source (Three-Phase)1/LConn1
  PMSM2/RConn2 -- Mechanical Rotational Reference3/LConn1
  Mjerenje kuta i brzine1/LConn1 -- Mechanical Rotational Reference2/LConn1 -- Ideal Torque Source2/RConn2 -- Mjerenje momenta1/RConn1 -- Ideal Torque Source2/LConn1
  Controlled Voltage Source (Three-Phase)2/RConn1 -- Mjerenje struje7/LConn1 -- Solver Configuration5/RConn1
  Simulink-PS Converter2/RConn1 -- Controlled Voltage Source (Three-Phase)2/LConn1
  Mjerenje struje7/RConn1 -- PMSM2/LConn1
  Electrical Reference1/LConn1 -- Controlled Voltage Source (Three-Phase)2/LConn2
  PMSM1/RConn2 -- Mechanical Rotational Reference15/LConn1
  PMSM2/RConn1 -- Mjerenje momenta1/LConn1
  Ideal Torque Source3/LConn1 -- Ideal Torque Source3/RConn2 -- Mechanical Rotational Reference1/LConn1 -- Mjerenje kuta i brzine2/LConn1 -- Mjerenje momenta2/RConn1
  Solver Configuration1/RConn1 -- Controlled Voltage Source (Three-Phase)3/RConn1 -- Mjerenje struje1/LConn1
  Electrical Reference2/LConn1 -- Controlled Voltage Source (Three-Phase)3/LConn2
  Mjerenje struje1/RConn1 -- PMSM3/LConn1
  PMSM3/RConn2 -- Mechanical Rotational Reference4/LConn1
  Simulink-PS Converter1/RConn1 -- Controlled Voltage Source (Three-Phase)3/LConn1
  PMSM3/RConn1 -- Mjerenje momenta2/LConn1
  Ideal Torque Source5/LConn1 -- Mechanical Rotational Reference7/LConn1 -- Ideal Torque Source5/RConn2 -- Mjerenje kuta i brzine4/LConn1 -- Mjerenje momenta4/RConn1
  Solver Configuration3/RConn1 -- Controlled Voltage Source (Three-Phase)5/RConn1 -- Mjerenje struje3/LConn1
  Electrical Reference4/LConn1 -- Controlled Voltage Source (Three-Phase)5/LConn2
  PMSM5/RConn2 -- Mechanical Rotational Reference8/LConn1
  PMSM5/RConn1 -- Mjerenje momenta4/LConn1
  Simulink-PS Converter4/RConn1 -- Controlled Voltage Source (Three-Phase)5/LConn1
  Mjerenje struje3/RConn1 -- PMSM5/LConn1
  Ideal Torque Source6/LConn1 -- Ideal Torque Source6/RConn2 -- Mechanical Rotational Reference9/LConn1 -- Mjerenje kuta i brzine5/LConn1 -- Mjerenje momenta5/RConn1
  Solver Configuration4/RConn1 -- Controlled Voltage Source (Three-Phase)6/RConn1 -- Mjerenje struje4/LConn1
  Electrical Reference5/LConn1 -- Controlled Voltage Source (Three-Phase)6/LConn2
  PMSM6/RConn2 -- Mechanical Rotational Reference10/LConn1
  PMSM6/RConn1 -- Mjerenje momenta5/LConn1
  Simulink-PS Converter5/RConn1 -- Controlled Voltage Source (Three-Phase)6/LConn1
  Mjerenje struje4/RConn1 -- PMSM6/LConn1
  Solver Configuration6/RConn1 -- Controlled Voltage Source (Three-Phase)7/RConn1 -- Mjerenje struje5/LConn1
  Electrical Reference6/LConn1 -- Controlled Voltage Source (Three-Phase)7/LConn2
  PMSM7/RConn2 -- Mechanical Rotational Reference12/LConn1
  PMSM7/RConn1 -- Mjerenje momenta6/LConn1
  Simulink-PS Converter6/RConn1 -- Controlled Voltage Source (Three-Phase)7/LConn1
  Mjerenje struje5/RConn1 -- PMSM7/LConn1
  Ideal Torque Source7/RConn2 -- Mechanical Rotational Reference11/LConn1
  Simulink-PS Converter/RConn1 -- Ideal Torque Source7/RConn1
  Mjerenje kuta i brzine6/LConn1 -- Inertia/LConn1 -- Ideal Torque Source7/LConn1 -- Mjerenje momenta6/RConn1

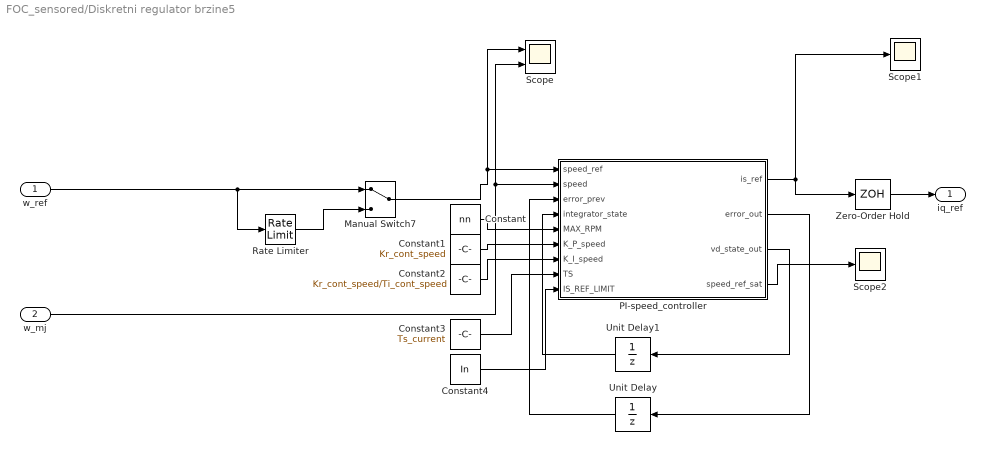
== system FOC_sensored/Diskretni regulator brzine5 ==
  w_ref : Inport
  w_mj : Inport  Port=2
  Constant : Constant  Value=nn  SampleTime=Ts_current
  Constant1 : Constant  Value=Kr_cont_speed  SampleTime=Ts_current
  Constant2 : Constant  Value=Kr_cont_speed/Ti_cont_speed  SampleTime=Ts_current
  Constant3 : Constant  Value=Ts_current  SampleTime=Ts_current
  Constant4 : Constant  Value=In  SampleTime=Ts_current
  Manual Switch7 : ManualSwitch
  PI-speed_controller : MATLAB Function  TreatAsAtomicUnit=on
  Rate Limiter : RateLimiter  RisingSlewLimit=Mn/J  FallingSlewLimit=-Mn/J  SampleTimeMode=inherited
  Scope : Scope  NumInputPorts=2
      settings: ActiveDisplayYMinimum=-62.500309400179823  ActiveDisplayYMaximum=562.50278460161849  DataLoggingVariableName=ScopeData4
  Scope1 : Scope
      settings: ActiveDisplayYMinimum=-62.5113191756852  ActiveDisplayYMaximum=70.802739564965421  DataLoggingVariableName=ScopeData5
  Scope2 : Scope
      settings: ActiveDisplayYMinimum=-1  ActiveDisplayYMaximum=1  DataLoggingVariableName=ScopeData10
  Unit Delay : UnitDelay  SampleTime=Ts_current
  Unit Delay1 : UnitDelay  SampleTime=Ts_current
  Zero-Order Hold : ZeroOrderHold  SampleTime=Ts_current
  iq_ref : Outport
  wires:
  Rate Limiter/1 -> Manual Switch7/2
  PI-speed_controller/2(error_out) -> Unit Delay/1
  Unit Delay/1 -> PI-speed_controller/3(error_prev)
  PI-speed_controller/3(vd_state_out) -> Unit Delay1/1
  Unit Delay1/1 -> PI-speed_controller/4(integrator_state)
  w_ref/1 -> Manual Switch7/1, Rate Limiter/1
  Manual Switch7/1 -> Scope/1, PI-speed_controller/1(speed_ref)
  w_mj/1 -> Scope/2, PI-speed_controller/2(speed)
  PI-speed_controller/1(is_ref) -> Scope1/1, Zero-Order Hold/1
  PI-speed_controller/4(speed_ref_sat) -> Scope2/1
  Zero-Order Hold/1 -> iq_ref/1
  Constant/1 -> PI-speed_controller/5(MAX_RPM)
  Constant1/1 -> PI-speed_controller/6(K_P_speed)
  Constant2/1 -> PI-speed_controller/7(K_I_speed)
  Constant3/1 -> PI-speed_controller/8(TS)
  Constant4/1 -> PI-speed_controller/9(IS_REF_LIMIT)

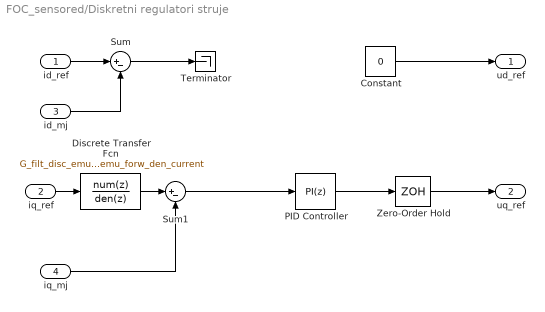
== system FOC_sensored/Diskretni regulatori struje ==
  id_ref : Inport
  iq_ref : Inport  Port=2
  id_mj : Inport  Port=3
  iq_mj : Inport  Port=4
  Constant : Constant  Value=0
  Discrete Transfer Fcn : DiscreteTransferFcn  Numerator=G_filt_disc_emu_forw_num_current  Denominator=G_filt_disc_emu_forw_den_current
  PID Controller : slpidlib/PID Controller  Controller=PI  Form=Ideal  TimeDomain=Discrete-time  UseExternalTs=off  SampleTime=-1  IntegratorMethod=Forward Euler  FilterMethod=Forward Euler  ControllerParametersSource=internal  P=Kr_cont_current  I=1/Ti_cont_current  UseKiTs=off  D=0  UseExternalDerivativeSource=off  N=100  UseFilter=on  TunerSelectOption=Transfer Function Based (PID Tuner App)  InitialConditionSource=internal  InitialConditionForIntegrator=0  InitialConditionForFilter=0  DifferentiatorICPrevScaledInput=0  ExternalReset=none  TrackingMode=off  Kt=1  LimitOutput=off  SatLimitsSource=internal  UpperSaturationLimit=inf  LowerSaturationLimit=-inf  LinearizeAsGain=on  AntiWindupMode=none  Kb=1  LimitIntegrator=off  UpperIntegratorSaturationLimit=inf  LowerIntegratorSaturationLimit=-inf  POutMin=[]  POutMax=[]  IOutMin=[]  IOutMax=[]  DOutMin=[]  DOutMax=[]  NOutMin=[]  NOutMax=[]  SumOutMin=[]  SumOutMax=[]  SaturationOutMin=[]  SaturationOutMax=[]  PParamMin=[]  PParamMax=[]  IParamMin=[]  IParamMax=[]  DParamMin=[]  DParamMax=[]  NParamMin=[]  NParamMax=[]  KbParamMin=[]  KbParamMax=[]  KtParamMin=[]  KtParamMax=[]  KbOutMin=[]  KbOutMax=[]  KtOutMin=[]  KtOutMax=[]  IntegratorOutMin=[]  IntegratorOutMax=[]  FilterOutMin=[]  FilterOutMax=[]  SumI1OutMin=[]  SumI1OutMax=[]  SumI2OutMin=[]  SumI2OutMax=[]  SumI3OutMin=[]  SumI3OutMax=[]  SumI4OutMin=[]  SumI4OutMax=[]  SumDOutMin=[]  SumDOutMax=[]  DifferentiatorOutMin=[]  DifferentiatorOutMax=[]  FilterDiffOutCoefMin=[]  FilterDiffOutCoefMax=[]  ReciprocalOutMin=[]  ReciprocalOutMax=[]  SumDenOutMin=[]  SumDenOutMax=[]  SumNumOutMin=[]  SumNumOutMax=[]  DivideOutMin=[]  DivideOutMax=[]  UdiffTsProdOutMin=[]  UdiffTsProdOutMax=[]  NTsProdOutMin=[]  NTsProdOutMax=[]  UintegralTsProdOutMin=[]  UintegralTsProdOutMax=[]  UngainTsProdOutMin=[]  UngainTsProdOutMax=[]  ClampingZeroOutDataTypeStr=Inherit: Inherit via back propagation  ClampingZeroOutMin=[]  ClampingZeroOutMax=[]  FilterDenConstantOutDataTypeStr=Inherit: Inherit via back propagation  FilterDenConstantOutMin=[]  FilterDenConstantOutMax=[]  PCopyOutDataTypeStr=Inherit: Inherit via back propagation  PCopyOutMin=[]  PCopyOutMax=[]  NCopyOutDataTypeStr=Inherit: Inherit via back propagation  NCopyOutMin=[]  NCopyOutMax=[]  IntegratorContinuousStateAttributes=''  IntegratorStateMustResolveToSignalObject=off  IntegratorRTWStateStorageClass=Auto  FilterContinuousStateAttributes=''  FilterStateMustResolveToSignalObject=off  FilterRTWStateStorageClass=Auto  ParallelPVariant=Passthrough  IdealPVariant=InternalParameters  IVariant=InternalParameters  DVariant=Disabled  IntegratorVariant=Discrete  SatVariant=Disabled  AWVariant=Passthrough  PCopyVariant=Disabled  TRVariant=Disabled  FdbkBlocksVariant=Forward  IdealPFdbkVariant=Disabled  SatFdbkVariant=Disabled  DerivativeFilterVariant=Disabled  NVariant=Disabled  NCopyVariant=Disabled_SignalSpec  FilterICVariant=Disabled  IntegratorICVariant=InternalICs  ExternalResetVariant=Disabled  TRSumVariant=Passthrough  SumFdbkVariant=Disabled  SumVariant=Sum_PI  TsampFilterVariant=InternalTs  TsampNgainVariant=Passthrough  TsampIntegralVariant=Disabled_SignalSpec  ExternalSaturationOutDataTypeStr=Inherit: Same as second input  DerivativeSourceVariant=Disabled  PreIntVariant=InternalPreInt
  Sum : Sum  Inputs=|+-
  Sum1 : Sum  Inputs=|+-
  Terminator : Terminator
  Zero-Order Hold : ZeroOrderHold  SampleTime=Ts_current
  ud_ref : Outport
  uq_ref : Outport  Port=2
  wires:
  id_ref/1 -> Sum/1
  id_mj/1 -> Sum/2
  Sum/1 -> Terminator/1
  Constant/1 -> ud_ref/1
  iq_mj/1 -> Sum1/2
  Sum1/1 -> PID Controller/1
  PID Controller/1 -> Zero-Order Hold/1
  Zero-Order Hold/1 -> uq_ref/1
  iq_ref/1 -> Discrete Transfer Fcn/1
  Discrete Transfer Fcn/1 -> Sum1/1
